simulink model "sample_kf"  (R2021a)
settings: Solver=VariableStepAuto  StartTime=0.0  StopTime=10.0  RelTol=1e-3
undefined symbols (not defined in the file or in its folder): Discrete, Time
libraries: simulink x2, ctrlSharedLib x2
settings Model: Creator=Willi  LastModifiedBy=Willi

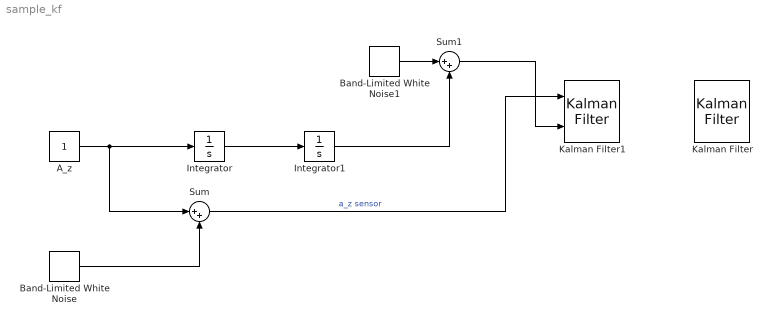
== system sample_kf ==
  A_z : Constant
  Band-Limited White Noise : simulink/Sources/Band-Limited White Noise  Cov=[0.1]  Ts=0.1  seed=[23341]
  Band-Limited White Noise1 : simulink/Sources/Band-Limited White Noise  Cov=[0.1]  Ts=0.1  seed=[23341]
  Integrator : Integrator
  Integrator1 : Integrator
  Kalman Filter : ctrlSharedLib/Kalman Filter  TimeDomain=Discrete-Time  UseCurrentEstimator=on  ModelSource=LTI State-Space Variable  ModelSourceVariable=ss(0.95,1,1,0,1)  A=0.95  B=1  C=1  D=0  NumberOfStates=1  NumberOfInputs=1  NumberOfOutputs=1  InitialEstimateSource=Dialog  X0=0  P0=10  UseK=off  UseGH=off  NumberOfProcessNoiseInputs=1  G=1  TimeInvariantG=on  H=0  TimeInvariantH=on  Q=0.05  TimeInvariantQ=on  R=1  TimeInvariantR=on  N=0  TimeInvariantN=on  AddInputPort=on  AddEnablePort=off  OutputEstimatedY=off  OutputP=off  Ts=-1
  Kalman Filter1 : ctrlSharedLib/Kalman Filter  TimeDomain=Discrete-Time  UseCurrentEstimator=on  ModelSource=LTI State-Space Variable  ModelSourceVariable=ss(0.95,1,1,0,1)  A=0.95  B=1  C=1  D=0  NumberOfStates=1  NumberOfInputs=1  NumberOfOutputs=1  InitialEstimateSource=Dialog  X0=0  P0=10  UseK=off  UseGH=off  NumberOfProcessNoiseInputs=1  G=1  TimeInvariantG=on  H=0  TimeInvariantH=on  Q=0.05  TimeInvariantQ=on  R=1  TimeInvariantR=on  N=0  TimeInvariantN=on  AddInputPort=on  AddEnablePort=off  OutputEstimatedY=off  OutputP=off  Ts=-1
  Sum : Sum  Inputs=|++
  Sum1 : Sum  Inputs=|++
  wires:
  Integrator/1 -> Integrator1/1
  A_z/1 -> Sum/1, Integrator/1
  Band-Limited White Noise/1 -> Sum/2
  Sum/1 -> Kalman Filter1/1  "a_z sensor"
  Band-Limited White Noise1/1 -> Sum1/1
  Integrator1/1 -> Sum1/2
  Sum1/1 -> Kalman Filter1/2
